simulink model "lead_compensator_with_user_defined_signal"  (R2023b)
settings: Solver=VariableStepAuto  StartTime=0.0  StopTime=20  RelTol=1e-3
undefined symbols (not defined in the file): sigbuilder_block
settings Model: Creator=kijun  LastModifiedBy=kijun

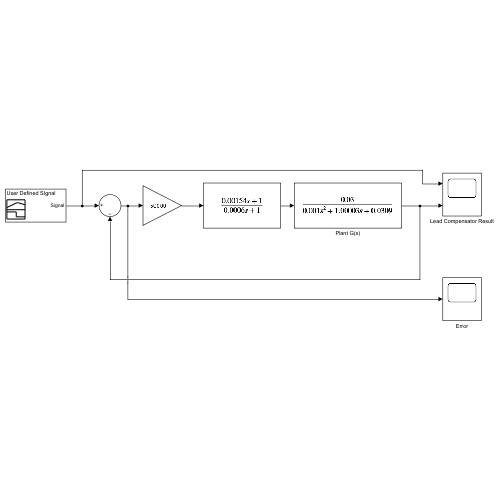
[thumbnail: Simulink's stored preview of the top-level diagram]
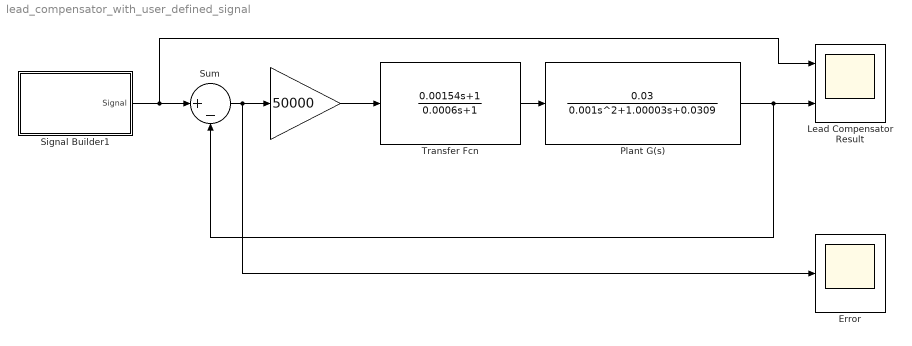
== system lead_compensator_with_user_defined_signal ==
  " " : Gain  Gain=50000
  Error : Scope
  Lead Compensator Result : Scope  NumInputPorts=2
  Plant G(s) : TransferFcn  Numerator=[0.03]  Denominator=[0.001 1.00003 0.0309]
  Signal Builder1 : Subsystem  Tag=STV Subsys  LoadFcn=sigbuilder_block('load');  StartFcn=sigbuilder_block('start');  StopFcn=sigbuilder_block('stop');  ClipboardFcn=sigbuilder_block('clipboard');  mask(Sigbuilder block){tuvar=[0:10]}
      mask help: Simulink:masks:SigbuilderBlock_MD
      mask init:
      | if ~strcmp(get_param(bdroot(gcbh),'SimulationStatus'),'stopped') tuvar = sigbuilder_block('maskInit'); end
      settings: CopyFcn=sigbuilder_block('copy');  DeleteFcn=sigbuilder_block('delete');  ModelCloseFcn=sigbuilder_block('modelClose');  PreSaveFcn=sigbuilder_block('preSave');  PauseFcn=sigbuilder_block('pause');  ContinueFcn=sigbuilder_block('continue');  NameChangeFcn=sigbuilder_block('namechange');  OpenFcn=sigbuilder_block('open',[282 66.6 823.2 453 ]);  CloseFcn=sigbuilder_block('close');
      mask Display: plot(0, 0, 100, 100,[2, 2, 32, 32, 2], [68, 8, 8, 68, 68],[32, 2], [38, 38], [32, 19, 2],[53, 60, 44], [32, 17, 17, 2],[16, 16, 31, 31]);txt = getActiveGroup(gcbh);text(2, 100, txt,'verticalAlignment', 'top');
  Sum : Sum  Inputs=|+-
  Transfer Fcn : TransferFcn  Numerator=[0.00154 1]  Denominator=[0.0006 1]
  wires:
  Plant G(s)/1 -> Lead Compensator Result/2, Sum/2
  " "/1 -> Transfer Fcn/1
  Signal Builder1/1(Signal) -> Lead Compensator Result/1, Sum/1
  Transfer Fcn/1 -> Plant G(s)/1
  Sum/1 -> Error/1, " "/1

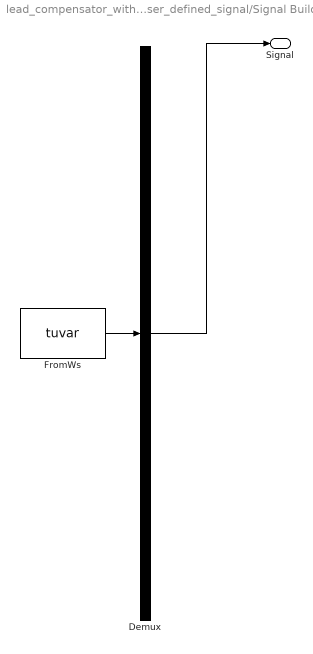
== system lead_compensator_with_user_defined_signal/Signal Builder1 ==
  Demux : Demux  Tag=STV Demux  Outputs=1
      settings: DisplayOption=none
  FromWs : FromWorkspace  Tag=STV FromWs  VariableName=tuvar
      SigBuilderData=|
      | common.afterFinalStr = 'Extrapolate'
      | common.sampleTime = 0
      | dataSet.timeRange = [0 14]
      | dataSet.name = 'User Defined SIgnal'
      | sbobj.Groups.Name = 'User Defined SIgnal'
      | sbobj.Groups.Signals.Name = 'Signal'
      | sbobj.Groups.Signals.XData = [0 3 8 11 14]
      | sbobj.Groups.Signals.YData = [0 63 63 0 0]
      | sbobj.Groups.TimeRange = [0 14]
  Signal : Outport  Tag=STV Outport
  wires:
  FromWs/1 -> Demux/1
  Demux/1 -> Signal/1
